simulink model "Linear_Kalman_filter1"  (R2025a)
settings: Solver=ode4  StartTime=0.0  StopTime=10.0  FixedStep=0.01  RelTol=1e-3
values from neighbouring files (symbols this model uses):
  Ac = [0,0,1,0 ... (first row only)    [init_linearization.m]
  Bc = [0,0 ... (first row only)    [init_linearization.m]
  Cc = [1,0,0,0;0,1,0,0]    [init_linearization.m]
  psi_op = pi/2    (= 1.57079632679)    [init_linearization.m]
  theta_op = -10*pi/180    (= -0.174532925199)    [init_linearization.m]
undefined symbols (not defined in the file or in its folder): L
settings Model: Creator=bulve  LastModifiedBy=BjørnErikUlveraker

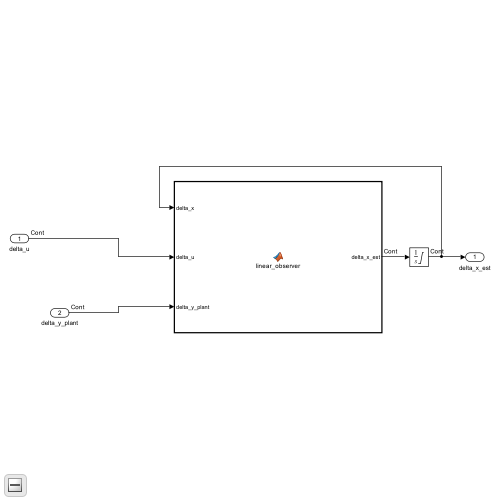
[thumbnail: Simulink's stored preview of the top-level diagram]
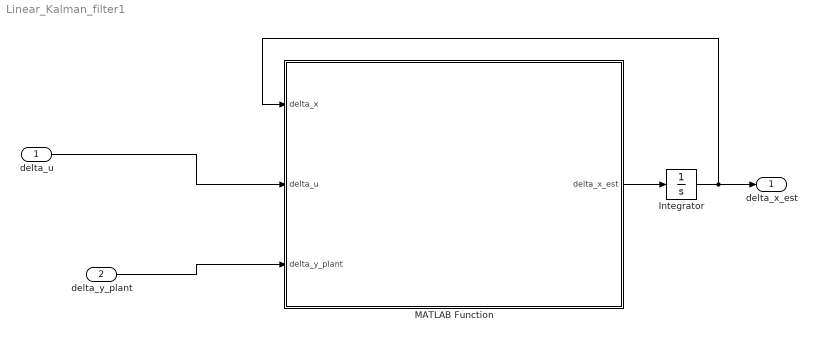
== system Linear_Kalman_filter1 ==
  delta_u : Inport
  delta_y_plant : Inport  Port=2
  Integrator : Integrator  LimitOutput=on  UpperSaturationLimit=[45*pi/180-theta_op;pi-psi_op;inf;inf]  LowerSaturationLimit=[-45*pi/180-theta_op;0-psi_op;-inf;-inf]
  MATLAB Function : MATLAB Function  TreatAsAtomicUnit=on
  delta_x_est : Outport
  wires:
  MATLAB Function/1(delta_x_est) -> Integrator/1
  Integrator/1 -> delta_x_est/1, MATLAB Function/1(delta_x)
  delta_u/1 -> MATLAB Function/2(delta_u)
  delta_y_plant/1 -> MATLAB Function/3(delta_y_plant)

== matlab function Linear_Kalman_filter1/MATLAB Function ==
  data: delta_x input size=[4 1]; delta_x_est output size=[4 1]; delta_u input size=[2 1]; delta_y_plant input size=[2 1]; Ac parameter size=[4 4]; Bc parameter size=[4 2]; Cc parameter size=[2 4]; L parameter
function delta_x_est = linear_observer(delta_x,delta_u,delta_y_plant, Ac, Bc, Cc, L)

delta_x = delta_x(:);
delta_u = delta_u(:);
delta_y_plant = delta_y_plant(:);


y_est = Cc*delta_x;

delta_x_est = Ac*delta_x +Bc*delta_u + L*(delta_y_plant-y_est);
